simulink model "W_server_mock_ClientServer_Model"  (R2024b)
settings: Solver=FixedStepDiscrete  StartTime=0.0  StopTime=10.0  FixedStep=0.05  RelTol=1e-3
settings Model: Tag=EP_AA_WRAPPER_SERVER_FUNCTIONS_MOCK  DataDictionary=Wrapper_ClientServer_Model.sldd  Creator=yatishc  LastModifiedBy=nabilekhoury
settings OptimizationCC: DefaultParameterBehavior=Inlined  EnhancedBackFolding=on  PassReuseOutputArgsAs=Individual arguments  ZeroExternalMemoryAtStartup=off  ZeroInternalMemoryAtStartup=off  OptimizeBlockOrder=speed  DifferentSizesBufferReuse=on  OptimizationCustomize=off  EfficientTunableParamExpr=on
settings DebuggingCC: ParameterTunabilityLossMsg=error
settings ModelReferenceCC: ModelReferenceNumInstancesAllowed=Single
settings SFSimCC: SimGenImportedTypeDefs=on  MATLABDynamicMemAlloc=off  SimTargetLang=C++
settings RTWCC: Description=Embedded Coder  SystemTargetFile=ert.tlc  GenCodeOnly=on  TemplateMakefile=ert_default_tmf  DataTypeReplacement=CDataTypesFixedWidth  TargetLang=C++
settings CodeAppCC: ForceParamTrailComments=on  IgnoreCustomStorageClasses=off  MaxIdLength=256  OperatorAnnotations=on  SimulinkDataObjDesc=on  SFDataObjDesc=on  CustomSymbolStrGlobalVar=w_$R$N$M  CustomSymbolStrType=w_$N$R$M_T  InsertBlockDesc=on
settings ERTTargetCC: TargetLangStandard=C++17 (ISO)  GenerateSampleERTMain=on  ERTCustomFileTemplate=example_file_process.tlc  MaxIdInt64=INT64_MAX  MinIdInt64=INT64_MIN  MaxIdUint64=UINT64_MAX  MaxIdInt32=INT32_MAX  MinIdInt32=INT32_MIN  MaxIdUint32=UINT32_MAX  MaxIdInt16=INT16_MAX  MinIdInt16=INT16_MIN  MaxIdUint16=UINT16_MAX  MaxIdInt8=INT8_MAX  MinIdInt8=INT8_MIN  MaxIdUint8=UINT8_MAX

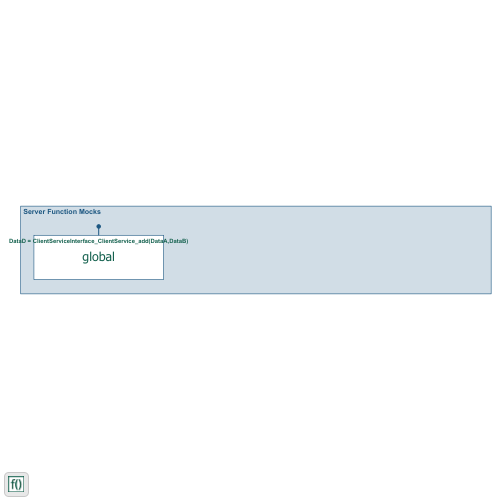
[thumbnail: Simulink's stored preview of the top-level diagram]
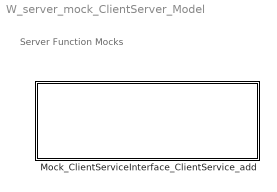
== system W_server_mock_ClientServer_Model ==
  note: Server Function Mocks
  Mock_ClientServiceInterface_ClientService_add : Subsystem  TreatAsAtomicUnit=on

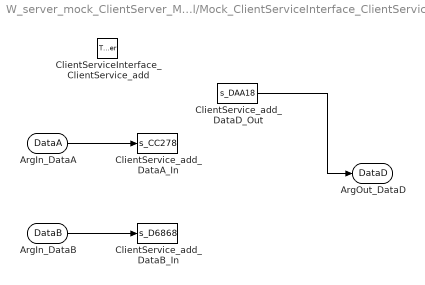
== system W_server_mock_ClientServer_Model/Mock_ClientServiceInterface_ClientService_add ==
  ClientServiceInterface_ClientService_add : TriggerPort  TriggerType=function-call  IsSimulinkFunction=on  FunctionName=ClientServiceInterface_ClientService_add  ScopeName=ClientService  VariantControl=(inherit)
  ClientService_add_DataA_In : DataStoreWrite  DataStoreName=s_CC278  IndexOptions=Index vector (dialog)  Indices=1  OutputSizes=1
  ClientService_add_DataB_In : DataStoreWrite  DataStoreName=s_D6868  IndexOptions=Index vector (dialog)  Indices=1  OutputSizes=1
  ClientService_add_DataD_Out : DataStoreRead  DataStoreName=s_DAA18  IndexOptions=Index vector (dialog)  Indices=1  OutputSizes=1
  ArgIn_DataA : ArgIn  PortDimensions=[1 1]  ArgumentName=DataA
  ArgIn_DataB : ArgIn  Port=2  PortDimensions=[1 1]  ArgumentName=DataB
  ArgOut_DataD : ArgOut  PortDimensions=[1 1]  ArgumentName=DataD
  wires:
  ArgIn_DataA/1 -> ClientService_add_DataA_In/1
  ArgIn_DataB/1 -> ClientService_add_DataB_In/1
  ClientService_add_DataD_Out/1 -> ArgOut_DataD/1
